simulink model "MBD_Discontinuities"  (R2021b)
settings: Solver=FixedStepAuto  StartTime=0.0  StopTime=10.0  RelTol=1e-3
libraries: simulink x2
settings Model: Creator=ADMIN  LastModifiedBy=ADMIN
settings OptimizationCC: DefaultParameterBehavior=Inlined  UseDivisionForNetSlopeComputation=on  GainParamInheritBuiltInType=on  UseFloatMulNetSlope=on  InlineInvariantSignals=on  PassReuseOutputArgsAs=Individual arguments  ZeroExternalMemoryAtStartup=off  ZeroInternalMemoryAtStartup=off  NoFixptDivByZeroProtection=on  EfficientFloat2IntCast=on  LifeSpan=1  OptimizeBlockOrder=speed  DifferentSizesBufferReuse=on  EfficientTunableParamExpr=on
settings DebuggingCC: ParameterTunabilityLossMsg=error  SFUnexpectedBacktrackingDiag=warning  SFNoUnconditionalDefaultTransitionDiag=warning
settings HardwareCC: ProdLongLongMode=on
settings SFSimCC: MATLABDynamicMemAlloc=off
settings RTWCC: Description=Embedded Coder  SystemTargetFile=ert.tlc  TemplateMakefile=ert_default_tmf  GenerateReport=on  BuildConfiguration=Debug  LaunchReport=on
settings CodeAppCC: ForceParamTrailComments=on  IgnoreCustomStorageClasses=off  OperatorAnnotations=on  SimulinkDataObjDesc=on  SFDataObjDesc=on  CustomSymbolStrGlobalVar=rt$N$M  CustomSymbolStrType=$N$M  CustomSymbolStrFcn=$N$M$F  CustomSymbolStrMacro=$N$M  InsertBlockDesc=on  EnableCustomComments=on
settings ERTTargetCC: TargetLangStandard=C99 (ISO)  GenerateSampleERTMain=on  IncludeMdlTerminateFcn=off  CombineSignalStateStructs=on  SupportComplex=off  SupportContinuousTime=on  InlinedParameterPlacement=NonHierarchical  ERTCustomFileTemplate=example_file_process.tlc  ERTFilePackagingFormat=CompactWithDataFile

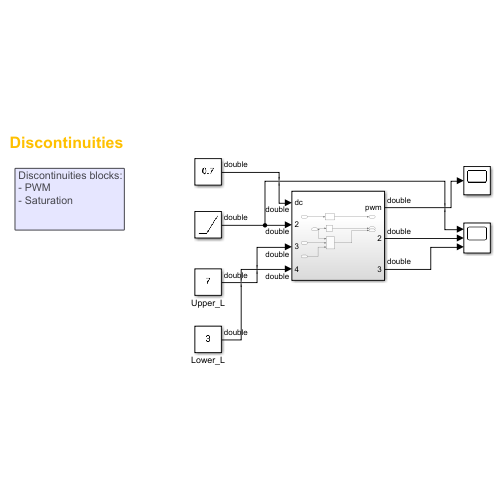
[thumbnail: Simulink's stored preview of the top-level diagram]
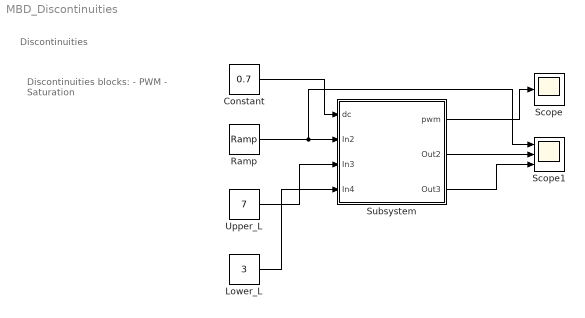
== system MBD_Discontinuities ==
  note: Discontinuities
  note: Discontinuities blocks:
      | - PWM
      | - Saturation
  Constant : Constant  Value=0.7
  Lower_L : Constant  Value=3
  Ramp : simulink/Sources/Ramp  slope=1  start=0  InitialOutput=0
  Scope : Scope
  Scope1 : Scope  NumInputPorts=3
  Subsystem : Subsystem
  Upper_L : Constant  Value=7
  wires:
  Ramp/1 -> Scope1/1, Subsystem/2(In2)
  Constant/1 -> Subsystem/1(dc)
  Upper_L/1 -> Subsystem/3(In3)
  Lower_L/1 -> Subsystem/4(In4)
  Subsystem/1(pwm) -> Scope/1
  Subsystem/2(Out2) -> Scope1/2
  Subsystem/3(Out3) -> Scope1/3

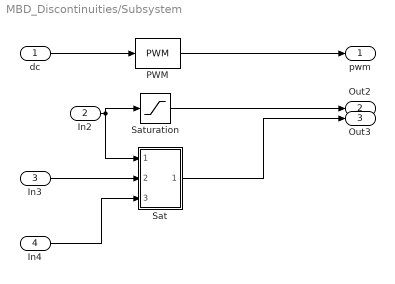
== system MBD_Discontinuities/Subsystem ==
  dc : Inport
  In2 : Inport  Port=2
  In3 : Inport  Port=3
  In4 : Inport  Port=4
  PWM : simulink/Discontinuities/PWM  DisableCoverage=on  Period=1  DisallowZeroDutyCycle=off  RunAtFixedTimeIntervals=on  SampleTime=0.001
  Sat : Subsystem
  Saturation : Saturate  UpperLimit=7  LowerLimit=3
  pwm : Outport
  Out2 : Outport  Port=2
  Out3 : Outport  Port=3
  wires:
  PWM/1 -> pwm/1
  In2/1 -> Sat/1(In1), Saturation/1
  In4/1 -> Sat/3(In3)
  dc/1 -> PWM/1
  In3/1 -> Sat/2(In2)
  Sat/1(Out1) -> Out3/1
  Saturation/1 -> Out2/1

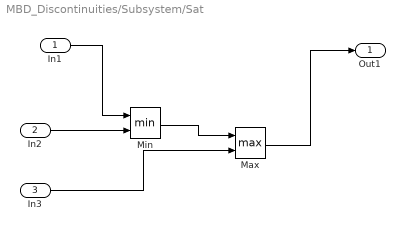
== system MBD_Discontinuities/Subsystem/Sat ==
  In1 : Inport
  In2 : Inport  Port=2
  In3 : Inport  Port=3
  Max : MinMax  Function=max  Inputs=2
  Min : MinMax  Inputs=2
  Out1 : Outport
  wires:
  Min/1 -> Max/1
  Max/1 -> Out1/1
  In1/1 -> Min/1
  In2/1 -> Min/2
  In3/1 -> Max/2
